simulink model "Hw03_P1_Spec2"  (R2024a)
settings: Solver=VariableStepAuto  StartTime=0.0  StopTime=10.0  RelTol=1e-3
model workspace (MAT data in the model file):
  Phi_n = 0
settings Model: Creator=bojack  LastModifiedBy=bojack
settings OptimizationCC: ReuseModelBlockBuffer=off
settings RTWCC: GPUComputeCapability=3.5

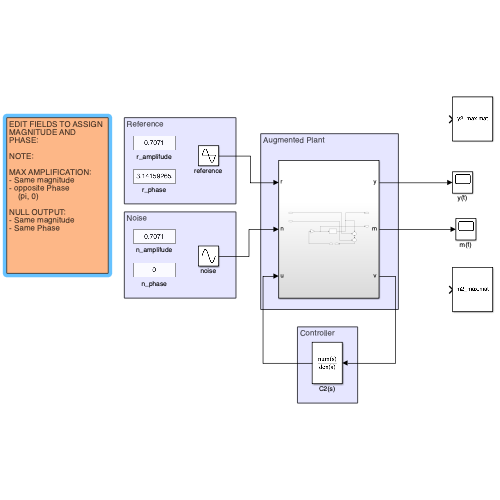
[thumbnail: Simulink's stored preview of the top-level diagram]
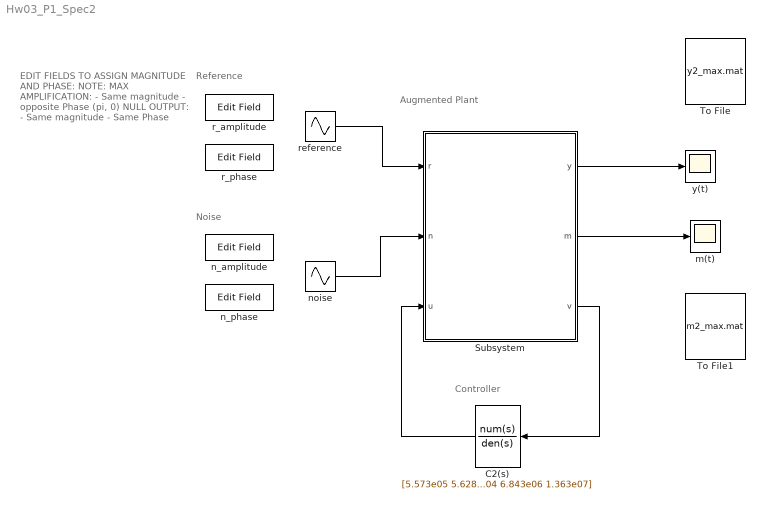
== system Hw03_P1_Spec2 ==
  note: EDIT FIELDS TO ASSIGN
      | MAGNITUDE AND
      | PHASE:
      |
      | NOTE:
      |
      | MAX AMPLIFICATION:
      | - Same magnitude
      | - opposite Phase
      |     (pi, 0)
      |
      | NULL OUTPUT:
      | - Same magnitude
      | - Same Phase
  note: Controller
  note: Augmented Plant
  note: Reference
  note: Noise
  C2(s) : TransferFcn  Numerator=[5.573e05 5.628e08 5.573e09]  Denominator=[1 1.463e04 6.843e06 1.363e07]
  Subsystem : Subsystem
  To File : ToFile  Filename=y2_max.mat  SaveFormat=Timeseries
  To File1 : ToFile  Filename=m2_max.mat  SaveFormat=Timeseries
  m(t) : Scope
  n_amplitude : EditField  LabelPosition=Hide  ShowInitialText=on  Alignment=Center
  n_phase : EditField  LabelPosition=Hide  ShowInitialText=on  Alignment=Center
  noise : Sin  Amplitude=0.7071  Frequency=10  SampleTime=0
  r_amplitude : EditField  LabelPosition=Hide  ShowInitialText=on  Alignment=Center
  r_phase : EditField  LabelPosition=Hide  ShowInitialText=on  Alignment=Center
  reference : Sin  Amplitude=0.7071  Frequency=10  Phase=pi  SampleTime=0
  y(t) : Scope
  wires:
  C2(s)/1 -> Subsystem/3(u)
  Subsystem/1(y) -> y(t)/1
  Subsystem/2(m) -> m(t)/1
  Subsystem/3(v) -> C2(s)/1
  reference/1 -> Subsystem/1(r)
  noise/1 -> Subsystem/2(n)

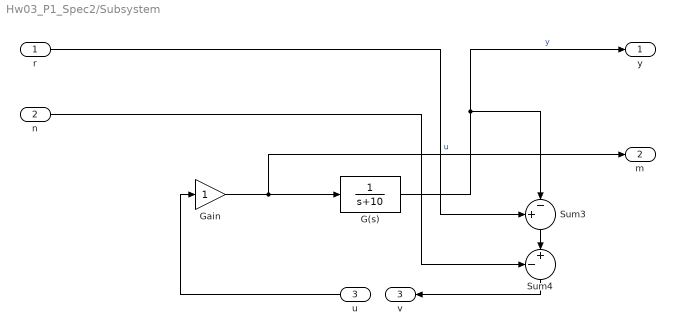
== system Hw03_P1_Spec2/Subsystem ==
  r : Inport
  n : Inport  Port=2
  u : Inport  Port=3
  G(s) : TransferFcn  Denominator=[1 10]
  Gain : Gain
  Sum3 : Sum  Inputs=+-|
  Sum4 : Sum  Inputs=-+|
  y : Outport
  m : Outport  Port=2
  v : Outport  Port=3
  wires:
  n/1 -> Sum4/1
  r/1 -> Sum3/1
  G(s)/1 -> y/1, Sum3/2  "y"
  u/1 -> Gain/1
  Gain/1 -> G(s)/1, m/1  "u"
  Sum3/1 -> Sum4/2
  Sum4/1 -> v/1
